simulink model "pocketcorr"  (Simulink 6.2)
settings: Solver=ode45  StartTime=0.0  StopTime=500  RelTol=1e-3
libraries: xbsIndex_r3 x44, xps_library x4, fft_library x4, pfb_library x4, correlator_library x1
settings Model: LastModifiedBy=dejesusc
settings DebuggingCC: SolverPrmCheckMsg=warning

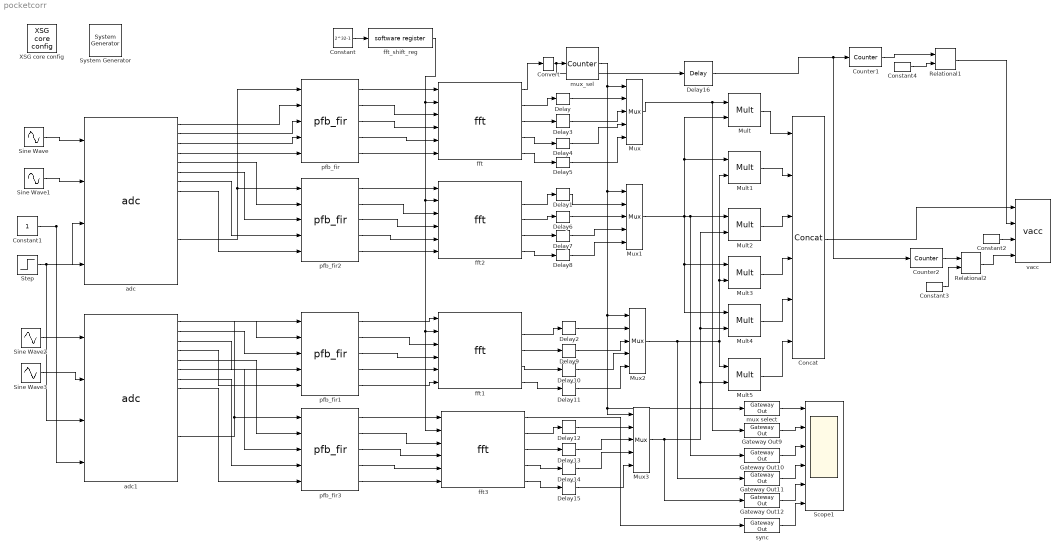
== system pocketcorr ==
  " System Generator" : xbsIndex_r3/ System Generator  Tag=genX  xilinxfamily=Virtex2P  part=xc2vp50  speed=-7  package=ff1152  synthesis_tool=XST  directory=./pocketcorr/sysgen  testbench=off  simulink_period=1  sysclk_period=3.9063  incr_netlist=off  trim_vbits=Everywhere in SubSystem  dbl_ovrd=According to Block Masks  core_generation=According to Block Masks  run_coregen=off  deprecated_control=off  eval_field=0
      settings: AttributesFormatString=System\nGenerator
  Concat : xbsIndex_r3/Concat  num_inputs=6  explicit_period=off  period=1  dbl_ovrd=off
  Constant : Constant  Value=2^32-1
  Constant1 : Constant
  Constant2 : xbsIndex_r3/Constant  const=0  equ=P=C  arith_type=Boolean  n_bits=1  bin_pt=0  opselect=C  inp2=PCIN>>17  opr=+  inp1=P  carry=CIN  iostate=0  explicit_period=on  period=1  dbl_ovrd=off
  Constant3 : xbsIndex_r3/Constant  const=32  equ=P=C  arith_type=Unsigned  n_bits=5  bin_pt=0  opselect=C  inp2=PCIN>>17  opr=+  inp1=P  carry=CIN  iostate=0  explicit_period=on  period=1  dbl_ovrd=off
  Constant4 : xbsIndex_r3/Constant  const=2^4  equ=P=C  arith_type=Unsigned  n_bits=5  bin_pt=0  opselect=C  inp2=PCIN>>17  opr=+  inp1=P  carry=CIN  iostate=0  explicit_period=on  period=1  dbl_ovrd=off
  Convert : xbsIndex_r3/Convert  arith_type=Boolean  n_bits=8  bin_pt=6  quantization=Truncate  overflow=Wrap  latency=0  explicit_period=off  period=1  dbl_ovrd=off  show_param=off  inserted_by_tool=off  pipeline=off
      settings: xl_area=[0, 0, 0, 0, 0, 0, 0]
  Counter1 : xbsIndex_r3/Counter  cnt_type=Free Running  n_bits=5  bin_pt=0  arith_type=Unsigned  start_count=0  cnt_to=Inf  cnt_by_val=1  operation=Up  explicit_period=off  period=1  load_pin=off  rst=on  en=off  dbl_ovrd=off  show_param=off  use_rpm=on  gen_core=off
      settings: xl_area=[0, 0, 0, 0, 0, 0, 0]
  Counter2 : xbsIndex_r3/Counter  cnt_type=Free Running  n_bits=20  bin_pt=0  arith_type=Unsigned  start_count=0  cnt_to=Inf  cnt_by_val=1  operation=Up  explicit_period=off  period=1  load_pin=off  rst=on  en=off  dbl_ovrd=off  show_param=off  use_rpm=on  gen_core=off
      settings: xl_area=[0, 0, 0, 0, 0, 0, 0]
  Delay{,1..2,12} (4 alike) : xbsIndex_r3/Delay  latency=4  reg_retiming=off  explicit_period=off  period=1  en=off  accept_only_valid=off  init_zero=on  dbl_ovrd=off  show_param=off
      settings: xl_area=[0, 0, 0, 0, 0, 0, 0]
  Delay{4,7,10,14} (4 alike) : xbsIndex_r3/Delay  latency=6  reg_retiming=off  explicit_period=off  period=1  en=off  accept_only_valid=off  init_zero=on  dbl_ovrd=off  show_param=off
      settings: xl_area=[0, 0, 0, 0, 0, 0, 0]
  Delay{5,8,11,15} (4 alike) : xbsIndex_r3/Delay  latency=7  reg_retiming=off  explicit_period=off  period=1  en=off  accept_only_valid=off  init_zero=on  dbl_ovrd=off  show_param=off
      settings: xl_area=[0, 0, 0, 0, 0, 0, 0]
  Delay{3,6,9,13} (4 alike) : xbsIndex_r3/Delay  latency=5  reg_retiming=off  explicit_period=off  period=1  en=off  accept_only_valid=off  init_zero=on  dbl_ovrd=off  show_param=off
      settings: xl_area=[0, 0, 0, 0, 0, 0, 0]
  Delay16 : xbsIndex_r3/Delay  latency=9  reg_retiming=off  explicit_period=off  period=1  en=off  accept_only_valid=off  init_zero=on  dbl_ovrd=off  show_param=off
      settings: xl_area=[0, 0, 0, 0, 0, 0, 0]
  Gateway Out{9..12} (4 alike) : xbsIndex_r3/Gateway Out  output_type=Double  nbits=8  bin_pt=6  arith_type=Boolean  quantization=Truncate  overflow=Wrap  hdl_port=on  timing_constraint=None  locs_specified=off  LOCs={}  needs_fixed_name=off  show_param=off
      settings: xl_area=[0, 0, 0, 0, 0, 0, 0]
  Mult{,1..5} (6 alike) : xbsIndex_r3/Mult  precision=Full  arith_type="Signed  (2's comp)"  n_bits=8  bin_pt=2  quantization=Truncate  overflow=Wrap  latency=5  explicit_period=off  period=1  en=off  dbl_ovrd=off  show_param=off  mult_type=Parallel  oversample=2  use_embedded=off  pipeline=on  use_rpm=on  placement_style=Rectangular Shape  gen_core=off
      settings: xl_area=[0, 0, 0, 0, 0, 0, 0]
  Mux{,1..3} (4 alike) : xbsIndex_r3/Mux  inputs=4  precision=Full  arith_type="Signed  (2's comp)"  n_bits=8  bin_pt=2  quantization=Truncate  overflow=Wrap  latency=0  explicit_period=off  period=1  en=off  dbl_ovrd=off  show_param=off  mux_type=off  use_rpm=off  gen_core=off
      settings: xl_area=[0, 0, 0, 0, 0, 0, 0]
  Relational1 : xbsIndex_r3/Relational  mode=a<b  latency=1  explicit_period=on  period=1  en=off  dbl_ovrd=off  show_param=off
      settings: xl_area=[0, 0, 0, 0, 0, 0, 0]
  Relational2 : xbsIndex_r3/Relational  mode=a<b  latency=1  explicit_period=on  period=1  en=off  dbl_ovrd=off  show_param=off
      settings: xl_area=[0, 0, 0, 0, 0, 0, 0]
  Scope1 : Scope  NumInputPorts=6
      settings: YMin=-5~-5~-5~-5~-5~-5  YMax=5~5~5~5~5~5
  Sine Wave : Sin  SampleTime=0
  Sine Wave1 : Sin  Phase=pi  SampleTime=0
  Sine Wave2 : Sin  Phase=pi/2  SampleTime=0
  Sine Wave3 : Sin  Phase=3*pi/2  SampleTime=0
  Step : Step  Time=10  Before=1  After=0  SampleTime=0
  XSG core config : xps_library/XSG core config  Tag=xps:xsg  hw_sys=iBOB  clk_src=adc0_clk  clk_rate=256  sample_period=1  probe_depth=512  mpc_type=powerpc405
  adc : xps_library/adc  Tag=xps:adc  adc_brd=iBOB:adc0  adc_clk_rate=1024  adc_interleave=off  sample_period=1
  adc1 : xps_library/adc  Tag=xps:adc  adc_brd=iBOB:adc1  adc_clk_rate=1024  adc_interleave=off  sample_period=1
  fft : fft_library/fft  FFTSize=5  BitWidth=18  n_inputs=2  quantization="Round  (unbiased: Even Values)"  overflow=Wrap  add_latency=2  mult_latency=3  bram_latency=2
      link override fft_biplex0/biplex_core/fft_stage_1/sync_delay_x/Constant: equ=P=C
      link override fft_biplex0/biplex_core/fft_stage_1/sync_delay_x/Constant1: equ=P=C
      link override fft_biplex0/biplex_core/fft_stage_1/sync_delay_x/Constant2: equ=P=C
      link override fft_biplex0/biplex_core/fft_stage_1/sync_delay_x/Constant3: equ=P=C
      link override fft_biplex0/biplex_core/fft_stage_2/sync_delay_x/Constant: equ=P=C
      link override fft_biplex0/biplex_core/fft_stage_2/sync_delay_x/Constant1: equ=P=C
      link override fft_biplex0/biplex_core/fft_stage_2/sync_delay_x/Constant2: equ=P=C
      link override fft_biplex0/biplex_core/fft_stage_2/sync_delay_x/Constant3: equ=P=C
      link override fft_biplex0/biplex_core/fft_stage_3/sync_delay_x/Constant: equ=P=C
      link override fft_biplex0/biplex_core/fft_stage_3/sync_delay_x/Constant1: equ=P=C
      link override fft_biplex0/biplex_core/fft_stage_3/sync_delay_x/Constant2: equ=P=C
      link override fft_biplex0/biplex_core/fft_stage_3/sync_delay_x/Constant3: equ=P=C
      link override fft_biplex0/biplex_core/fft_stage_4/sync_delay_x/Constant: equ=P=C
      link override fft_biplex0/biplex_core/fft_stage_4/sync_delay_x/Constant1: equ=P=C
      link override fft_biplex0/biplex_core/fft_stage_4/sync_delay_x/Constant2: equ=P=C
      link override fft_biplex0/biplex_core/fft_stage_4/sync_delay_x/Constant3: equ=P=C
      link override fft_biplex0/biplex_core/fft_stage_5/sync_delay_x/Constant: equ=P=C
      link override fft_biplex0/biplex_core/fft_stage_5/sync_delay_x/Constant1: equ=P=C
      link override fft_biplex0/biplex_core/fft_stage_5/sync_delay_x/Constant2: equ=P=C
      link override fft_biplex0/biplex_core/fft_stage_5/sync_delay_x/Constant3: equ=P=C
      link override fft_biplex0/biplex_core/fft_stage_6/sync_delay_x/Constant: equ=P=C
      link override fft_biplex0/biplex_core/fft_stage_6/sync_delay_x/Constant1: equ=P=C
      link override fft_biplex0/biplex_core/fft_stage_6/sync_delay_x/Constant2: equ=P=C
      link override fft_biplex0/biplex_core/fft_stage_6/sync_delay_x/Constant3: equ=P=C
      link override fft_biplex0/biplex_core/fft_stage_7/sync_delay_x/Constant: equ=P=C
      link override fft_biplex0/biplex_core/fft_stage_7/sync_delay_x/Constant1: equ=P=C
      link override fft_biplex0/biplex_core/fft_stage_7/sync_delay_x/Constant2: equ=P=C
      link override fft_biplex0/biplex_core/fft_stage_7/sync_delay_x/Constant3: equ=P=C
      link override fft_biplex0/biplex_cplx_unscrambler/delay_bram1/Constant2: equ=P=C
      link override fft_biplex0/biplex_cplx_unscrambler/reorder/Constant: equ=P=C
      link override fft_biplex0/biplex_cplx_unscrambler/reorder/sync_delay/Constant: equ=P=C
      link override fft_biplex0/biplex_cplx_unscrambler/reorder/sync_delay/Constant1: equ=P=C
      link override fft_biplex0/biplex_cplx_unscrambler/reorder/sync_delay/Constant2: equ=P=C
      link override fft_biplex0/biplex_cplx_unscrambler/reorder/sync_delay/Constant3: equ=P=C
      link override fft_biplex0/biplex_cplx_unscrambler/reorder1/Constant: equ=P=C
      link override fft_biplex0/biplex_cplx_unscrambler/reorder1/sync_delay/Constant: equ=P=C
      link override fft_biplex0/biplex_cplx_unscrambler/reorder1/sync_delay/Constant1: equ=P=C
      link override fft_biplex0/biplex_cplx_unscrambler/reorder1/sync_delay/Constant2: equ=P=C
      link override fft_biplex0/biplex_cplx_unscrambler/reorder1/sync_delay/Constant3: equ=P=C
      link override fft_biplex0/biplex_cplx_unscrambler/sync_delay/Constant: equ=P=C
      link override fft_biplex0/biplex_cplx_unscrambler/sync_delay/Constant1: equ=P=C
      link override fft_biplex0/biplex_cplx_unscrambler/sync_delay/Constant2: equ=P=C
      link override fft_biplex0/biplex_cplx_unscrambler/sync_delay/Constant3: equ=P=C
      link override fft_biplex1/biplex_core/fft_stage_1/sync_delay_x/Constant: equ=P=C
      link override fft_biplex1/biplex_core/fft_stage_1/sync_delay_x/Constant1: equ=P=C
      link override fft_biplex1/biplex_core/fft_stage_1/sync_delay_x/Constant2: equ=P=C
      link override fft_biplex1/biplex_core/fft_stage_1/sync_delay_x/Constant3: equ=P=C
      link override fft_biplex1/biplex_core/fft_stage_2/sync_delay_x/Constant: equ=P=C
      link override fft_biplex1/biplex_core/fft_stage_2/sync_delay_x/Constant1: equ=P=C
      link override fft_biplex1/biplex_core/fft_stage_2/sync_delay_x/Constant2: equ=P=C
      link override fft_biplex1/biplex_core/fft_stage_2/sync_delay_x/Constant3: equ=P=C
      link override fft_biplex1/biplex_core/fft_stage_3/sync_delay_x/Constant: equ=P=C
      link override fft_biplex1/biplex_core/fft_stage_3/sync_delay_x/Constant1: equ=P=C
      link override fft_biplex1/biplex_core/fft_stage_3/sync_delay_x/Constant2: equ=P=C
      link override fft_biplex1/biplex_core/fft_stage_3/sync_delay_x/Constant3: equ=P=C
      link override fft_biplex1/biplex_core/fft_stage_4/sync_delay_x/Constant: equ=P=C
      link override fft_biplex1/biplex_core/fft_stage_4/sync_delay_x/Constant1: equ=P=C
      link override fft_biplex1/biplex_core/fft_stage_4/sync_delay_x/Constant2: equ=P=C
      link override fft_biplex1/biplex_core/fft_stage_4/sync_delay_x/Constant3: equ=P=C
      link override fft_biplex1/biplex_core/fft_stage_5/sync_delay_x/Constant: equ=P=C
      link override fft_biplex1/biplex_core/fft_stage_5/sync_delay_x/Constant1: equ=P=C
      link override fft_biplex1/biplex_core/fft_stage_5/sync_delay_x/Constant2: equ=P=C
      link override fft_biplex1/biplex_core/fft_stage_5/sync_delay_x/Constant3: equ=P=C
      link override fft_biplex1/biplex_core/fft_stage_6/sync_delay_x/Constant: equ=P=C
      link override fft_biplex1/biplex_core/fft_stage_6/sync_delay_x/Constant1: equ=P=C
      link override fft_biplex1/biplex_core/fft_stage_6/sync_delay_x/Constant2: equ=P=C
      link override fft_biplex1/biplex_core/fft_stage_6/sync_delay_x/Constant3: equ=P=C
      link override fft_biplex1/biplex_core/fft_stage_7/sync_delay_x/Constant: equ=P=C
      link override fft_biplex1/biplex_core/fft_stage_7/sync_delay_x/Constant1: equ=P=C
      link override fft_biplex1/biplex_core/fft_stage_7/sync_delay_x/Constant2: equ=P=C
      link override fft_biplex1/biplex_core/fft_stage_7/sync_delay_x/Constant3: equ=P=C
      link override fft_biplex1/biplex_cplx_unscrambler/delay_bram1/Constant2: equ=P=C
      link override fft_biplex1/biplex_cplx_unscrambler/reorder/Constant: equ=P=C
      link override fft_biplex1/biplex_cplx_unscrambler/reorder/sync_delay/Constant: equ=P=C
      link override fft_biplex1/biplex_cplx_unscrambler/reorder/sync_delay/Constant1: equ=P=C
      link override fft_biplex1/biplex_cplx_unscrambler/reorder/sync_delay/Constant2: equ=P=C
      link override fft_biplex1/biplex_cplx_unscrambler/reorder/sync_delay/Constant3: equ=P=C
      link override fft_biplex1/biplex_cplx_unscrambler/reorder1/Constant: equ=P=C
      link override fft_biplex1/biplex_cplx_unscrambler/reorder1/sync_delay/Constant: equ=P=C
      link override fft_biplex1/biplex_cplx_unscrambler/reorder1/sync_delay/Constant1: equ=P=C
      link override fft_biplex1/biplex_cplx_unscrambler/reorder1/sync_delay/Constant2: equ=P=C
      link override fft_biplex1/biplex_cplx_unscrambler/reorder1/sync_delay/Constant3: equ=P=C
      link override fft_biplex1/biplex_cplx_unscrambler/sync_delay/Constant: equ=P=C
      link override fft_biplex1/biplex_cplx_unscrambler/sync_delay/Constant1: equ=P=C
      link override fft_biplex1/biplex_cplx_unscrambler/sync_delay/Constant2: equ=P=C
      link override fft_biplex1/biplex_cplx_unscrambler/sync_delay/Constant3: equ=P=C
      link override fft_unscrambler/Constant: const=1  equ=P=C  arith_type=Boolean  explicit_period=on
      link override fft_unscrambler/sync_delay/Constant: equ=P=C
      link override fft_unscrambler/sync_delay/Constant1: equ=P=C
      link override fft_unscrambler/sync_delay/Constant2: equ=P=C
      link override fft_unscrambler/sync_delay/Constant3: equ=P=C
  fft1 : fft_library/fft  FFTSize=5  BitWidth=18  n_inputs=2  quantization="Round  (unbiased: Even Values)"  overflow=Wrap  add_latency=2  mult_latency=3  bram_latency=2
      link override fft_biplex0/biplex_core/fft_stage_1/sync_delay_x/Constant: equ=P=C
      link override fft_biplex0/biplex_core/fft_stage_1/sync_delay_x/Constant1: equ=P=C
      link override fft_biplex0/biplex_core/fft_stage_1/sync_delay_x/Constant2: equ=P=C
      link override fft_biplex0/biplex_core/fft_stage_1/sync_delay_x/Constant3: equ=P=C
      link override fft_biplex0/biplex_core/fft_stage_2/sync_delay_x/Constant: equ=P=C
      link override fft_biplex0/biplex_core/fft_stage_2/sync_delay_x/Constant1: equ=P=C
      link override fft_biplex0/biplex_core/fft_stage_2/sync_delay_x/Constant2: equ=P=C
      link override fft_biplex0/biplex_core/fft_stage_2/sync_delay_x/Constant3: equ=P=C
      link override fft_biplex0/biplex_core/fft_stage_3/sync_delay_x/Constant: equ=P=C
      link override fft_biplex0/biplex_core/fft_stage_3/sync_delay_x/Constant1: equ=P=C
      link override fft_biplex0/biplex_core/fft_stage_3/sync_delay_x/Constant2: equ=P=C
      link override fft_biplex0/biplex_core/fft_stage_3/sync_delay_x/Constant3: equ=P=C
      link override fft_biplex0/biplex_core/fft_stage_4/sync_delay_x/Constant: equ=P=C
      link override fft_biplex0/biplex_core/fft_stage_4/sync_delay_x/Constant1: equ=P=C
      link override fft_biplex0/biplex_core/fft_stage_4/sync_delay_x/Constant2: equ=P=C
      link override fft_biplex0/biplex_core/fft_stage_4/sync_delay_x/Constant3: equ=P=C
      link override fft_biplex0/biplex_core/fft_stage_5/sync_delay_x/Constant: equ=P=C
      link override fft_biplex0/biplex_core/fft_stage_5/sync_delay_x/Constant1: equ=P=C
      link override fft_biplex0/biplex_core/fft_stage_5/sync_delay_x/Constant2: equ=P=C
      link override fft_biplex0/biplex_core/fft_stage_5/sync_delay_x/Constant3: equ=P=C
      link override fft_biplex0/biplex_core/fft_stage_6/sync_delay_x/Constant: equ=P=C
      link override fft_biplex0/biplex_core/fft_stage_6/sync_delay_x/Constant1: equ=P=C
      link override fft_biplex0/biplex_core/fft_stage_6/sync_delay_x/Constant2: equ=P=C
      link override fft_biplex0/biplex_core/fft_stage_6/sync_delay_x/Constant3: equ=P=C
      link override fft_biplex0/biplex_core/fft_stage_7/sync_delay_x/Constant: equ=P=C
      link override fft_biplex0/biplex_core/fft_stage_7/sync_delay_x/Constant1: equ=P=C
      link override fft_biplex0/biplex_core/fft_stage_7/sync_delay_x/Constant2: equ=P=C
      link override fft_biplex0/biplex_core/fft_stage_7/sync_delay_x/Constant3: equ=P=C
      link override fft_biplex0/biplex_cplx_unscrambler/delay_bram1/Constant2: equ=P=C
      link override fft_biplex0/biplex_cplx_unscrambler/reorder/Constant: equ=P=C
      link override fft_biplex0/biplex_cplx_unscrambler/reorder/sync_delay/Constant: equ=P=C
      link override fft_biplex0/biplex_cplx_unscrambler/reorder/sync_delay/Constant1: equ=P=C
      link override fft_biplex0/biplex_cplx_unscrambler/reorder/sync_delay/Constant2: equ=P=C
      link override fft_biplex0/biplex_cplx_unscrambler/reorder/sync_delay/Constant3: equ=P=C
      link override fft_biplex0/biplex_cplx_unscrambler/reorder1/Constant: equ=P=C
      link override fft_biplex0/biplex_cplx_unscrambler/reorder1/sync_delay/Constant: equ=P=C
      link override fft_biplex0/biplex_cplx_unscrambler/reorder1/sync_delay/Constant1: equ=P=C
      link override fft_biplex0/biplex_cplx_unscrambler/reorder1/sync_delay/Constant2: equ=P=C
      link override fft_biplex0/biplex_cplx_unscrambler/reorder1/sync_delay/Constant3: equ=P=C
      link override fft_biplex0/biplex_cplx_unscrambler/sync_delay/Constant: equ=P=C
      link override fft_biplex0/biplex_cplx_unscrambler/sync_delay/Constant1: equ=P=C
      link override fft_biplex0/biplex_cplx_unscrambler/sync_delay/Constant2: equ=P=C
      link override fft_biplex0/biplex_cplx_unscrambler/sync_delay/Constant3: equ=P=C
      link override fft_biplex1/biplex_core/fft_stage_1/sync_delay_x/Constant: equ=P=C
      link override fft_biplex1/biplex_core/fft_stage_1/sync_delay_x/Constant1: equ=P=C
      link override fft_biplex1/biplex_core/fft_stage_1/sync_delay_x/Constant2: equ=P=C
      link override fft_biplex1/biplex_core/fft_stage_1/sync_delay_x/Constant3: equ=P=C
      link override fft_biplex1/biplex_core/fft_stage_2/sync_delay_x/Constant: equ=P=C
      link override fft_biplex1/biplex_core/fft_stage_2/sync_delay_x/Constant1: equ=P=C
      link override fft_biplex1/biplex_core/fft_stage_2/sync_delay_x/Constant2: equ=P=C
      link override fft_biplex1/biplex_core/fft_stage_2/sync_delay_x/Constant3: equ=P=C
      link override fft_biplex1/biplex_core/fft_stage_3/sync_delay_x/Constant: equ=P=C
      link override fft_biplex1/biplex_core/fft_stage_3/sync_delay_x/Constant1: equ=P=C
      link override fft_biplex1/biplex_core/fft_stage_3/sync_delay_x/Constant2: equ=P=C
      link override fft_biplex1/biplex_core/fft_stage_3/sync_delay_x/Constant3: equ=P=C
      link override fft_biplex1/biplex_core/fft_stage_4/sync_delay_x/Constant: equ=P=C
      link override fft_biplex1/biplex_core/fft_stage_4/sync_delay_x/Constant1: equ=P=C
      link override fft_biplex1/biplex_core/fft_stage_4/sync_delay_x/Constant2: equ=P=C
      link override fft_biplex1/biplex_core/fft_stage_4/sync_delay_x/Constant3: equ=P=C
      link override fft_biplex1/biplex_core/fft_stage_5/sync_delay_x/Constant: equ=P=C
      link override fft_biplex1/biplex_core/fft_stage_5/sync_delay_x/Constant1: equ=P=C
      link override fft_biplex1/biplex_core/fft_stage_5/sync_delay_x/Constant2: equ=P=C
      link override fft_biplex1/biplex_core/fft_stage_5/sync_delay_x/Constant3: equ=P=C
      link override fft_biplex1/biplex_core/fft_stage_6/sync_delay_x/Constant: equ=P=C
      link override fft_biplex1/biplex_core/fft_stage_6/sync_delay_x/Constant1: equ=P=C
      link override fft_biplex1/biplex_core/fft_stage_6/sync_delay_x/Constant2: equ=P=C
      link override fft_biplex1/biplex_core/fft_stage_6/sync_delay_x/Constant3: equ=P=C
      link override fft_biplex1/biplex_core/fft_stage_7/sync_delay_x/Constant: equ=P=C
      link override fft_biplex1/biplex_core/fft_stage_7/sync_delay_x/Constant1: equ=P=C
      link override fft_biplex1/biplex_core/fft_stage_7/sync_delay_x/Constant2: equ=P=C
      link override fft_biplex1/biplex_core/fft_stage_7/sync_delay_x/Constant3: equ=P=C
      link override fft_biplex1/biplex_cplx_unscrambler/delay_bram1/Constant2: equ=P=C
      link override fft_biplex1/biplex_cplx_unscrambler/reorder/Constant: equ=P=C
      link override fft_biplex1/biplex_cplx_unscrambler/reorder/sync_delay/Constant: equ=P=C
      link override fft_biplex1/biplex_cplx_unscrambler/reorder/sync_delay/Constant1: equ=P=C
      link override fft_biplex1/biplex_cplx_unscrambler/reorder/sync_delay/Constant2: equ=P=C
      link override fft_biplex1/biplex_cplx_unscrambler/reorder/sync_delay/Constant3: equ=P=C
      link override fft_biplex1/biplex_cplx_unscrambler/reorder1/Constant: equ=P=C
      link override fft_biplex1/biplex_cplx_unscrambler/reorder1/sync_delay/Constant: equ=P=C
      link override fft_biplex1/biplex_cplx_unscrambler/reorder1/sync_delay/Constant1: equ=P=C
      link override fft_biplex1/biplex_cplx_unscrambler/reorder1/sync_delay/Constant2: equ=P=C
      link override fft_biplex1/biplex_cplx_unscrambler/reorder1/sync_delay/Constant3: equ=P=C
      link override fft_biplex1/biplex_cplx_unscrambler/sync_delay/Constant: equ=P=C
      link override fft_biplex1/biplex_cplx_unscrambler/sync_delay/Constant1: equ=P=C
      link override fft_biplex1/biplex_cplx_unscrambler/sync_delay/Constant2: equ=P=C
      link override fft_biplex1/biplex_cplx_unscrambler/sync_delay/Constant3: equ=P=C
      link override fft_unscrambler/Constant: equ=P=C  const=1  arith_type=Boolean  explicit_period=on
      link override fft_unscrambler/sync_delay/Constant: equ=P=C
      link override fft_unscrambler/sync_delay/Constant1: equ=P=C
      link override fft_unscrambler/sync_delay/Constant2: equ=P=C
      link override fft_unscrambler/sync_delay/Constant3: equ=P=C
  fft2 : fft_library/fft  FFTSize=5  BitWidth=18  n_inputs=2  quantization="Round  (unbiased: Even Values)"  overflow=Wrap  add_latency=2  mult_latency=3  bram_latency=2
      link override fft_biplex0/biplex_core/fft_stage_1/sync_delay_x/Constant: equ=P=C
      link override fft_biplex0/biplex_core/fft_stage_1/sync_delay_x/Constant1: equ=P=C
      link override fft_biplex0/biplex_core/fft_stage_1/sync_delay_x/Constant2: equ=P=C
      link override fft_biplex0/biplex_core/fft_stage_1/sync_delay_x/Constant3: equ=P=C
      link override fft_biplex0/biplex_core/fft_stage_2/sync_delay_x/Constant: equ=P=C
      link override fft_biplex0/biplex_core/fft_stage_2/sync_delay_x/Constant1: equ=P=C
      link override fft_biplex0/biplex_core/fft_stage_2/sync_delay_x/Constant2: equ=P=C
      link override fft_biplex0/biplex_core/fft_stage_2/sync_delay_x/Constant3: equ=P=C
      link override fft_biplex0/biplex_core/fft_stage_3/sync_delay_x/Constant: equ=P=C
      link override fft_biplex0/biplex_core/fft_stage_3/sync_delay_x/Constant1: equ=P=C
      link override fft_biplex0/biplex_core/fft_stage_3/sync_delay_x/Constant2: equ=P=C
      link override fft_biplex0/biplex_core/fft_stage_3/sync_delay_x/Constant3: equ=P=C
      link override fft_biplex0/biplex_core/fft_stage_4/sync_delay_x/Constant: equ=P=C
      link override fft_biplex0/biplex_core/fft_stage_4/sync_delay_x/Constant1: equ=P=C
      link override fft_biplex0/biplex_core/fft_stage_4/sync_delay_x/Constant2: equ=P=C
      link override fft_biplex0/biplex_core/fft_stage_4/sync_delay_x/Constant3: equ=P=C
      link override fft_biplex0/biplex_core/fft_stage_5/sync_delay_x/Constant: equ=P=C
      link override fft_biplex0/biplex_core/fft_stage_5/sync_delay_x/Constant1: equ=P=C
      link override fft_biplex0/biplex_core/fft_stage_5/sync_delay_x/Constant2: equ=P=C
      link override fft_biplex0/biplex_core/fft_stage_5/sync_delay_x/Constant3: equ=P=C
      link override fft_biplex0/biplex_core/fft_stage_6/sync_delay_x/Constant: equ=P=C
      link override fft_biplex0/biplex_core/fft_stage_6/sync_delay_x/Constant1: equ=P=C
      link override fft_biplex0/biplex_core/fft_stage_6/sync_delay_x/Constant2: equ=P=C
      link override fft_biplex0/biplex_core/fft_stage_6/sync_delay_x/Constant3: equ=P=C
      link override fft_biplex0/biplex_core/fft_stage_7/sync_delay_x/Constant: equ=P=C
      link override fft_biplex0/biplex_core/fft_stage_7/sync_delay_x/Constant1: equ=P=C
      link override fft_biplex0/biplex_core/fft_stage_7/sync_delay_x/Constant2: equ=P=C
      link override fft_biplex0/biplex_core/fft_stage_7/sync_delay_x/Constant3: equ=P=C
      link override fft_biplex0/biplex_cplx_unscrambler/delay_bram1/Constant2: equ=P=C
      link override fft_biplex0/biplex_cplx_unscrambler/reorder/Constant: equ=P=C
      link override fft_biplex0/biplex_cplx_unscrambler/reorder/sync_delay/Constant: equ=P=C
      link override fft_biplex0/biplex_cplx_unscrambler/reorder/sync_delay/Constant1: equ=P=C
      link override fft_biplex0/biplex_cplx_unscrambler/reorder/sync_delay/Constant2: equ=P=C
      link override fft_biplex0/biplex_cplx_unscrambler/reorder/sync_delay/Constant3: equ=P=C
      link override fft_biplex0/biplex_cplx_unscrambler/reorder1/Constant: equ=P=C
      link override fft_biplex0/biplex_cplx_unscrambler/reorder1/sync_delay/Constant: equ=P=C
      link override fft_biplex0/biplex_cplx_unscrambler/reorder1/sync_delay/Constant1: equ=P=C
      link override fft_biplex0/biplex_cplx_unscrambler/reorder1/sync_delay/Constant2: equ=P=C
      link override fft_biplex0/biplex_cplx_unscrambler/reorder1/sync_delay/Constant3: equ=P=C
      link override fft_biplex0/biplex_cplx_unscrambler/sync_delay/Constant: equ=P=C
      link override fft_biplex0/biplex_cplx_unscrambler/sync_delay/Constant1: equ=P=C
      link override fft_biplex0/biplex_cplx_unscrambler/sync_delay/Constant2: equ=P=C
      link override fft_biplex0/biplex_cplx_unscrambler/sync_delay/Constant3: equ=P=C
      link override fft_biplex1/biplex_core/fft_stage_1/sync_delay_x/Constant: equ=P=C
      link override fft_biplex1/biplex_core/fft_stage_1/sync_delay_x/Constant1: equ=P=C
      link override fft_biplex1/biplex_core/fft_stage_1/sync_delay_x/Constant2: equ=P=C
      link override fft_biplex1/biplex_core/fft_stage_1/sync_delay_x/Constant3: equ=P=C
      link override fft_biplex1/biplex_core/fft_stage_2/sync_delay_x/Constant: equ=P=C
      link override fft_biplex1/biplex_core/fft_stage_2/sync_delay_x/Constant1: equ=P=C
      link override fft_biplex1/biplex_core/fft_stage_2/sync_delay_x/Constant2: equ=P=C
      link override fft_biplex1/biplex_core/fft_stage_2/sync_delay_x/Constant3: equ=P=C
      link override fft_biplex1/biplex_core/fft_stage_3/sync_delay_x/Constant: equ=P=C
      link override fft_biplex1/biplex_core/fft_stage_3/sync_delay_x/Constant1: equ=P=C
      link override fft_biplex1/biplex_core/fft_stage_3/sync_delay_x/Constant2: equ=P=C
      link override fft_biplex1/biplex_core/fft_stage_3/sync_delay_x/Constant3: equ=P=C
      link override fft_biplex1/biplex_core/fft_stage_4/sync_delay_x/Constant: equ=P=C
      link override fft_biplex1/biplex_core/fft_stage_4/sync_delay_x/Constant1: equ=P=C
      link override fft_biplex1/biplex_core/fft_stage_4/sync_delay_x/Constant2: equ=P=C
      link override fft_biplex1/biplex_core/fft_stage_4/sync_delay_x/Constant3: equ=P=C
      link override fft_biplex1/biplex_core/fft_stage_5/sync_delay_x/Constant: equ=P=C
      link override fft_biplex1/biplex_core/fft_stage_5/sync_delay_x/Constant1: equ=P=C
      link override fft_biplex1/biplex_core/fft_stage_5/sync_delay_x/Constant2: equ=P=C
      link override fft_biplex1/biplex_core/fft_stage_5/sync_delay_x/Constant3: equ=P=C
      link override fft_biplex1/biplex_core/fft_stage_6/sync_delay_x/Constant: equ=P=C
      link override fft_biplex1/biplex_core/fft_stage_6/sync_delay_x/Constant1: equ=P=C
      link override fft_biplex1/biplex_core/fft_stage_6/sync_delay_x/Constant2: equ=P=C
      link override fft_biplex1/biplex_core/fft_stage_6/sync_delay_x/Constant3: equ=P=C
      link override fft_biplex1/biplex_core/fft_stage_7/sync_delay_x/Constant: equ=P=C
      link override fft_biplex1/biplex_core/fft_stage_7/sync_delay_x/Constant1: equ=P=C
      link override fft_biplex1/biplex_core/fft_stage_7/sync_delay_x/Constant2: equ=P=C
      link override fft_biplex1/biplex_core/fft_stage_7/sync_delay_x/Constant3: equ=P=C
      link override fft_biplex1/biplex_cplx_unscrambler/delay_bram1/Constant2: equ=P=C
      link override fft_biplex1/biplex_cplx_unscrambler/reorder/Constant: equ=P=C
      link override fft_biplex1/biplex_cplx_unscrambler/reorder/sync_delay/Constant: equ=P=C
      link override fft_biplex1/biplex_cplx_unscrambler/reorder/sync_delay/Constant1: equ=P=C
      link override fft_biplex1/biplex_cplx_unscrambler/reorder/sync_delay/Constant2: equ=P=C
      link override fft_biplex1/biplex_cplx_unscrambler/reorder/sync_delay/Constant3: equ=P=C
      link override fft_biplex1/biplex_cplx_unscrambler/reorder1/Constant: equ=P=C
      link override fft_biplex1/biplex_cplx_unscrambler/reorder1/sync_delay/Constant: equ=P=C
      link override fft_biplex1/biplex_cplx_unscrambler/reorder1/sync_delay/Constant1: equ=P=C
      link override fft_biplex1/biplex_cplx_unscrambler/reorder1/sync_delay/Constant2: equ=P=C
      link override fft_biplex1/biplex_cplx_unscrambler/reorder1/sync_delay/Constant3: equ=P=C
      link override fft_biplex1/biplex_cplx_unscrambler/sync_delay/Constant: equ=P=C
      link override fft_biplex1/biplex_cplx_unscrambler/sync_delay/Constant1: equ=P=C
      link override fft_biplex1/biplex_cplx_unscrambler/sync_delay/Constant2: equ=P=C
      link override fft_biplex1/biplex_cplx_unscrambler/sync_delay/Constant3: equ=P=C
      link override fft_unscrambler/Constant: equ=P=C  const=1  arith_type=Boolean  explicit_period=on
      link override fft_unscrambler/sync_delay/Constant: equ=P=C
      link override fft_unscrambler/sync_delay/Constant1: equ=P=C
      link override fft_unscrambler/sync_delay/Constant2: equ=P=C
      link override fft_unscrambler/sync_delay/Constant3: equ=P=C
  fft3 : fft_library/fft  FFTSize=5  BitWidth=18  n_inputs=2  quantization="Round  (unbiased: Even Values)"  overflow=Wrap  add_latency=2  mult_latency=3  bram_latency=2
      link override fft_biplex0/biplex_core/fft_stage_1/sync_delay_x/Constant: equ=P=C
      link override fft_biplex0/biplex_core/fft_stage_1/sync_delay_x/Constant1: equ=P=C
      link override fft_biplex0/biplex_core/fft_stage_1/sync_delay_x/Constant2: equ=P=C
      link override fft_biplex0/biplex_core/fft_stage_1/sync_delay_x/Constant3: equ=P=C
      link override fft_biplex0/biplex_core/fft_stage_2/sync_delay_x/Constant: equ=P=C
      link override fft_biplex0/biplex_core/fft_stage_2/sync_delay_x/Constant1: equ=P=C
      link override fft_biplex0/biplex_core/fft_stage_2/sync_delay_x/Constant2: equ=P=C
      link override fft_biplex0/biplex_core/fft_stage_2/sync_delay_x/Constant3: equ=P=C
      link override fft_biplex0/biplex_core/fft_stage_3/sync_delay_x/Constant: equ=P=C
      link override fft_biplex0/biplex_core/fft_stage_3/sync_delay_x/Constant1: equ=P=C
      link override fft_biplex0/biplex_core/fft_stage_3/sync_delay_x/Constant2: equ=P=C
      link override fft_biplex0/biplex_core/fft_stage_3/sync_delay_x/Constant3: equ=P=C
      link override fft_biplex0/biplex_core/fft_stage_4/sync_delay_x/Constant: equ=P=C
      link override fft_biplex0/biplex_core/fft_stage_4/sync_delay_x/Constant1: equ=P=C
      link override fft_biplex0/biplex_core/fft_stage_4/sync_delay_x/Constant2: equ=P=C
      link override fft_biplex0/biplex_core/fft_stage_4/sync_delay_x/Constant3: equ=P=C
      link override fft_biplex0/biplex_core/fft_stage_5/sync_delay_x/Constant: equ=P=C
      link override fft_biplex0/biplex_core/fft_stage_5/sync_delay_x/Constant1: equ=P=C
      link override fft_biplex0/biplex_core/fft_stage_5/sync_delay_x/Constant2: equ=P=C
      link override fft_biplex0/biplex_core/fft_stage_5/sync_delay_x/Constant3: equ=P=C
      link override fft_biplex0/biplex_core/fft_stage_6/sync_delay_x/Constant: equ=P=C
      link override fft_biplex0/biplex_core/fft_stage_6/sync_delay_x/Constant1: equ=P=C
      link override fft_biplex0/biplex_core/fft_stage_6/sync_delay_x/Constant2: equ=P=C
      link override fft_biplex0/biplex_core/fft_stage_6/sync_delay_x/Constant3: equ=P=C
      link override fft_biplex0/biplex_core/fft_stage_7/sync_delay_x/Constant: equ=P=C
      link override fft_biplex0/biplex_core/fft_stage_7/sync_delay_x/Constant1: equ=P=C
      link override fft_biplex0/biplex_core/fft_stage_7/sync_delay_x/Constant2: equ=P=C
      link override fft_biplex0/biplex_core/fft_stage_7/sync_delay_x/Constant3: equ=P=C
      link override fft_biplex0/biplex_cplx_unscrambler/delay_bram1/Constant2: equ=P=C
      link override fft_biplex0/biplex_cplx_unscrambler/reorder/Constant: equ=P=C
      link override fft_biplex0/biplex_cplx_unscrambler/reorder/sync_delay/Constant: equ=P=C
      link override fft_biplex0/biplex_cplx_unscrambler/reorder/sync_delay/Constant1: equ=P=C
      link override fft_biplex0/biplex_cplx_unscrambler/reorder/sync_delay/Constant2: equ=P=C
      link override fft_biplex0/biplex_cplx_unscrambler/reorder/sync_delay/Constant3: equ=P=C
      link override fft_biplex0/biplex_cplx_unscrambler/reorder1/Constant: equ=P=C
      link override fft_biplex0/biplex_cplx_unscrambler/reorder1/sync_delay/Constant: equ=P=C
      link override fft_biplex0/biplex_cplx_unscrambler/reorder1/sync_delay/Constant1: equ=P=C
      link override fft_biplex0/biplex_cplx_unscrambler/reorder1/sync_delay/Constant2: equ=P=C
      link override fft_biplex0/biplex_cplx_unscrambler/reorder1/sync_delay/Constant3: equ=P=C
      link override fft_biplex0/biplex_cplx_unscrambler/sync_delay/Constant: equ=P=C
      link override fft_biplex0/biplex_cplx_unscrambler/sync_delay/Constant1: equ=P=C
      link override fft_biplex0/biplex_cplx_unscrambler/sync_delay/Constant2: equ=P=C
      link override fft_biplex0/biplex_cplx_unscrambler/sync_delay/Constant3: equ=P=C
      link override fft_biplex1/biplex_core/fft_stage_1/sync_delay_x/Constant: equ=P=C
      link override fft_biplex1/biplex_core/fft_stage_1/sync_delay_x/Constant1: equ=P=C
      link override fft_biplex1/biplex_core/fft_stage_1/sync_delay_x/Constant2: equ=P=C
      link override fft_biplex1/biplex_core/fft_stage_1/sync_delay_x/Constant3: equ=P=C
      link override fft_biplex1/biplex_core/fft_stage_2/sync_delay_x/Constant: equ=P=C
      link override fft_biplex1/biplex_core/fft_stage_2/sync_delay_x/Constant1: equ=P=C
      link override fft_biplex1/biplex_core/fft_stage_2/sync_delay_x/Constant2: equ=P=C
      link override fft_biplex1/biplex_core/fft_stage_2/sync_delay_x/Constant3: equ=P=C
      link override fft_biplex1/biplex_core/fft_stage_3/sync_delay_x/Constant: equ=P=C
      link override fft_biplex1/biplex_core/fft_stage_3/sync_delay_x/Constant1: equ=P=C
      link override fft_biplex1/biplex_core/fft_stage_3/sync_delay_x/Constant2: equ=P=C
      link override fft_biplex1/biplex_core/fft_stage_3/sync_delay_x/Constant3: equ=P=C
      link override fft_biplex1/biplex_core/fft_stage_4/sync_delay_x/Constant: equ=P=C
      link override fft_biplex1/biplex_core/fft_stage_4/sync_delay_x/Constant1: equ=P=C
      link override fft_biplex1/biplex_core/fft_stage_4/sync_delay_x/Constant2: equ=P=C
      link override fft_biplex1/biplex_core/fft_stage_4/sync_delay_x/Constant3: equ=P=C
      link override fft_biplex1/biplex_core/fft_stage_5/sync_delay_x/Constant: equ=P=C
      link override fft_biplex1/biplex_core/fft_stage_5/sync_delay_x/Constant1: equ=P=C
      link override fft_biplex1/biplex_core/fft_stage_5/sync_delay_x/Constant2: equ=P=C
      link override fft_biplex1/biplex_core/fft_stage_5/sync_delay_x/Constant3: equ=P=C
      link override fft_biplex1/biplex_core/fft_stage_6/sync_delay_x/Constant: equ=P=C
      link override fft_biplex1/biplex_core/fft_stage_6/sync_delay_x/Constant1: equ=P=C
      link override fft_biplex1/biplex_core/fft_stage_6/sync_delay_x/Constant2: equ=P=C
      link override fft_biplex1/biplex_core/fft_stage_6/sync_delay_x/Constant3: equ=P=C
      link override fft_biplex1/biplex_core/fft_stage_7/sync_delay_x/Constant: equ=P=C
      link override fft_biplex1/biplex_core/fft_stage_7/sync_delay_x/Constant1: equ=P=C
      link override fft_biplex1/biplex_core/fft_stage_7/sync_delay_x/Constant2: equ=P=C
      link override fft_biplex1/biplex_core/fft_stage_7/sync_delay_x/Constant3: equ=P=C
      link override fft_biplex1/biplex_cplx_unscrambler/delay_bram1/Constant2: equ=P=C
      link override fft_biplex1/biplex_cplx_unscrambler/reorder/Constant: equ=P=C
      link override fft_biplex1/biplex_cplx_unscrambler/reorder/sync_delay/Constant: equ=P=C
      link override fft_biplex1/biplex_cplx_unscrambler/reorder/sync_delay/Constant1: equ=P=C
      link override fft_biplex1/biplex_cplx_unscrambler/reorder/sync_delay/Constant2: equ=P=C
      link override fft_biplex1/biplex_cplx_unscrambler/reorder/sync_delay/Constant3: equ=P=C
      link override fft_biplex1/biplex_cplx_unscrambler/reorder1/Constant: equ=P=C
      link override fft_biplex1/biplex_cplx_unscrambler/reorder1/sync_delay/Constant: equ=P=C
      link override fft_biplex1/biplex_cplx_unscrambler/reorder1/sync_delay/Constant1: equ=P=C
      link override fft_biplex1/biplex_cplx_unscrambler/reorder1/sync_delay/Constant2: equ=P=C
      link override fft_biplex1/biplex_cplx_unscrambler/reorder1/sync_delay/Constant3: equ=P=C
      link override fft_biplex1/biplex_cplx_unscrambler/sync_delay/Constant: equ=P=C
      link override fft_biplex1/biplex_cplx_unscrambler/sync_delay/Constant1: equ=P=C
      link override fft_biplex1/biplex_cplx_unscrambler/sync_delay/Constant2: equ=P=C
      link override fft_biplex1/biplex_cplx_unscrambler/sync_delay/Constant3: equ=P=C
      link override fft_unscrambler/Constant: equ=P=C  const=1  arith_type=Boolean  explicit_period=on
      link override fft_unscrambler/sync_delay/Constant: equ=P=C
      link override fft_unscrambler/sync_delay/Constant1: equ=P=C
      link override fft_unscrambler/sync_delay/Constant2: equ=P=C
      link override fft_unscrambler/sync_delay/Constant3: equ=P=C
  fft_shift_reg : xps_library/software register  Tag=xps:sw_reg  io_dir=From Processor  arith_type=Unsigned  bitwidth=32  bin_pt=0  sample_period=1  gw_name=pocketcorr_fft_shift_reg_user_data_out
  mux select : xbsIndex_r3/Gateway Out  output_type=Double  nbits=8  bin_pt=6  arith_type=Boolean  quantization=Truncate  overflow=Wrap  hdl_port=on  timing_constraint=None  locs_specified=off  LOCs={}  needs_fixed_name=off  show_param=off
      settings: xl_area=[0, 0, 0, 0, 0, 0, 0]
  mux_sel : xbsIndex_r3/Counter  cnt_type=Free Running  n_bits=2  bin_pt=0  arith_type=Unsigned  start_count=0  cnt_to=3  cnt_by_val=1  operation=Up  explicit_period=off  period=1  load_pin=off  rst=on  en=off  dbl_ovrd=off  show_param=off  use_rpm=on  gen_core=off
      settings: xl_area=[0, 0, 0, 0, 0, 0, 0]
  pfb_fir : pfb_library/pfb_fir  PFBSize=5  TotalTaps=2  WindowType=hamming  n_inputs=2  MakeBiplex=off  BitWidthIn=8  BitWidthOut=18  CoeffBitWidth=8  CoeffDistMem=off  add_latency=2  mult_latency=3  bram_latency=2  quantization="Round  (unbiased: +/- Inf)"  fwidth=1
      link override pol1_in1_first_tap/sync_delay/Constant: equ=P=C
      link override pol1_in1_first_tap/sync_delay/Constant1: equ=P=C
      link override pol1_in1_first_tap/sync_delay/Constant2: equ=P=C
      link override pol1_in1_first_tap/sync_delay/Constant3: equ=P=C
      link override pol1_in2_first_tap/sync_delay/Constant: equ=P=C
      link override pol1_in2_first_tap/sync_delay/Constant1: equ=P=C
      link override pol1_in2_first_tap/sync_delay/Constant2: equ=P=C
      link override pol1_in2_first_tap/sync_delay/Constant3: equ=P=C
      link override pol1_in3_first_tap/sync_delay/Constant: equ=P=C
      link override pol1_in3_first_tap/sync_delay/Constant1: equ=P=C
      link override pol1_in3_first_tap/sync_delay/Constant2: equ=P=C
      link override pol1_in3_first_tap/sync_delay/Constant3: equ=P=C
      link override pol1_in4_first_tap/sync_delay/Constant: equ=P=C
      link override pol1_in4_first_tap/sync_delay/Constant1: equ=P=C
      link override pol1_in4_first_tap/sync_delay/Constant2: equ=P=C
      link override pol1_in4_first_tap/sync_delay/Constant3: equ=P=C
  pfb_fir1 : pfb_library/pfb_fir  PFBSize=5  TotalTaps=2  WindowType=hamming  n_inputs=2  MakeBiplex=off  BitWidthIn=8  BitWidthOut=18  CoeffBitWidth=8  CoeffDistMem=off  add_latency=2  mult_latency=3  bram_latency=2  quantization="Round  (unbiased: +/- Inf)"  fwidth=1
      link override pol1_in1_first_tap/sync_delay/Constant: equ=P=C
      link override pol1_in1_first_tap/sync_delay/Constant1: equ=P=C
      link override pol1_in1_first_tap/sync_delay/Constant2: equ=P=C
      link override pol1_in1_first_tap/sync_delay/Constant3: equ=P=C
      link override pol1_in2_first_tap/sync_delay/Constant: equ=P=C
      link override pol1_in2_first_tap/sync_delay/Constant1: equ=P=C
      link override pol1_in2_first_tap/sync_delay/Constant2: equ=P=C
      link override pol1_in2_first_tap/sync_delay/Constant3: equ=P=C
      link override pol1_in3_first_tap/sync_delay/Constant: equ=P=C
      link override pol1_in3_first_tap/sync_delay/Constant1: equ=P=C
      link override pol1_in3_first_tap/sync_delay/Constant2: equ=P=C
      link override pol1_in3_first_tap/sync_delay/Constant3: equ=P=C
      link override pol1_in4_first_tap/sync_delay/Constant: equ=P=C
      link override pol1_in4_first_tap/sync_delay/Constant1: equ=P=C
      link override pol1_in4_first_tap/sync_delay/Constant2: equ=P=C
      link override pol1_in4_first_tap/sync_delay/Constant3: equ=P=C
  pfb_fir2 : pfb_library/pfb_fir  PFBSize=5  TotalTaps=2  WindowType=hamming  n_inputs=2  MakeBiplex=off  BitWidthIn=8  BitWidthOut=18  CoeffBitWidth=8  CoeffDistMem=off  add_latency=2  mult_latency=3  bram_latency=2  quantization="Round  (unbiased: +/- Inf)"  fwidth=1
      link override pol1_in1_first_tap/sync_delay/Constant: equ=P=C
      link override pol1_in1_first_tap/sync_delay/Constant1: equ=P=C
      link override pol1_in1_first_tap/sync_delay/Constant2: equ=P=C
      link override pol1_in1_first_tap/sync_delay/Constant3: equ=P=C
      link override pol1_in2_first_tap/sync_delay/Constant: equ=P=C
      link override pol1_in2_first_tap/sync_delay/Constant1: equ=P=C
      link override pol1_in2_first_tap/sync_delay/Constant2: equ=P=C
      link override pol1_in2_first_tap/sync_delay/Constant3: equ=P=C
      link override pol1_in3_first_tap/sync_delay/Constant: equ=P=C
      link override pol1_in3_first_tap/sync_delay/Constant1: equ=P=C
      link override pol1_in3_first_tap/sync_delay/Constant2: equ=P=C
      link override pol1_in3_first_tap/sync_delay/Constant3: equ=P=C
      link override pol1_in4_first_tap/sync_delay/Constant: equ=P=C
      link override pol1_in4_first_tap/sync_delay/Constant1: equ=P=C
      link override pol1_in4_first_tap/sync_delay/Constant2: equ=P=C
      link override pol1_in4_first_tap/sync_delay/Constant3: equ=P=C
  pfb_fir3 : pfb_library/pfb_fir  PFBSize=5  TotalTaps=2  WindowType=hamming  n_inputs=2  MakeBiplex=off  BitWidthIn=8  BitWidthOut=18  CoeffBitWidth=8  CoeffDistMem=off  add_latency=2  mult_latency=3  bram_latency=2  quantization="Round  (unbiased: +/- Inf)"  fwidth=1
      link override pol1_in1_first_tap/sync_delay/Constant: equ=P=C
      link override pol1_in1_first_tap/sync_delay/Constant1: equ=P=C
      link override pol1_in1_first_tap/sync_delay/Constant2: equ=P=C
      link override pol1_in1_first_tap/sync_delay/Constant3: equ=P=C
      link override pol1_in2_first_tap/sync_delay/Constant: equ=P=C
      link override pol1_in2_first_tap/sync_delay/Constant1: equ=P=C
      link override pol1_in2_first_tap/sync_delay/Constant2: equ=P=C
      link override pol1_in2_first_tap/sync_delay/Constant3: equ=P=C
      link override pol1_in3_first_tap/sync_delay/Constant: equ=P=C
      link override pol1_in3_first_tap/sync_delay/Constant1: equ=P=C
      link override pol1_in3_first_tap/sync_delay/Constant2: equ=P=C
      link override pol1_in3_first_tap/sync_delay/Constant3: equ=P=C
      link override pol1_in4_first_tap/sync_delay/Constant: equ=P=C
      link override pol1_in4_first_tap/sync_delay/Constant1: equ=P=C
      link override pol1_in4_first_tap/sync_delay/Constant2: equ=P=C
      link override pol1_in4_first_tap/sync_delay/Constant3: equ=P=C
  sync : xbsIndex_r3/Gateway Out  output_type=Double  nbits=8  bin_pt=6  arith_type=Boolean  quantization=Truncate  overflow=Wrap  hdl_port=on  timing_constraint=None  locs_specified=off  LOCs={}  needs_fixed_name=off  show_param=off
      settings: xl_area=[0, 0, 0, 0, 0, 0, 0]
  vacc : correlator_library/vacc  vlen=32/2-6  n_bits=32  bin_pt=0  add_latency=2  arith_type=Unsigned  BitWidthIn=36  BinPtIn=35  streams=6
      link override acc_core/const0: equ=P=C
      link override acc_core/const1: equ=P=C
      link override acc_core/vacc_fifo1/constant: equ=P=C
  wires:
  adc/13 -> pfb_fir/1, pfb_fir2/1
  pfb_fir/1 -> fft/1
  pfb_fir/2 -> fft/3
  pfb_fir/3 -> fft/4
  fft_shift_reg/1 -> fft/2, fft2/2, fft1/2, fft3/2
  Constant/1 -> fft_shift_reg/1
  pfb_fir/4 -> fft/5
  pfb_fir/5 -> fft/6
  adc/1 -> pfb_fir/2
  adc/2 -> pfb_fir/3
  adc/3 -> pfb_fir/4
  adc/4 -> pfb_fir/5
  pfb_fir1/1 -> fft1/1
  pfb_fir1/2 -> fft1/3
  pfb_fir1/3 -> fft1/4
  pfb_fir1/4 -> fft1/5
  pfb_fir1/5 -> fft1/6
  pfb_fir3/1 -> fft3/1
  pfb_fir3/2 -> fft3/3
  pfb_fir3/3 -> fft3/4
  pfb_fir3/4 -> fft3/5
  pfb_fir3/5 -> fft3/6
  adc1/13 -> pfb_fir1/1, pfb_fir3/1
  adc1/1 -> pfb_fir1/2
  adc1/2 -> pfb_fir1/3
  adc1/3 -> pfb_fir1/4
  adc1/4 -> pfb_fir1/5
  adc1/5 -> pfb_fir3/2
  adc1/6 -> pfb_fir3/3
  adc1/7 -> pfb_fir3/4
  adc1/8 -> pfb_fir3/5
  pfb_fir2/1 -> fft2/1
  pfb_fir2/2 -> fft2/3
  pfb_fir2/3 -> fft2/4
  pfb_fir2/4 -> fft2/5
  pfb_fir2/5 -> fft2/6
  adc/5 -> pfb_fir2/2
  adc/6 -> pfb_fir2/3
  adc/7 -> pfb_fir2/4
  adc/8 -> pfb_fir2/5
  Constant1/1 -> adc/4, adc1/4
  fft/2 -> Delay/1
  fft2/2 -> Delay1/1
  fft1/2 -> Delay2/1
  fft3/2 -> Delay12/1
  fft/3 -> Delay3/1
  fft/4 -> Delay4/1
  fft/5 -> Delay5/1
  Mux/1 -> Mult/1, Gateway Out9/1
  Delay/1 -> Mux/2
  Delay3/1 -> Mux/3
  Delay4/1 -> Mux/4
  Delay5/1 -> Mux/5
  mux_sel/1 -> Mux/1, Mux1/1, Mux2/1, Mux3/1, mux select/1
  Delay1/1 -> Mux1/2
  Mux1/1 -> Mult/2, Mult1/1, Mult3/1, Mult4/1, Mult2/1, Gateway Out10/1
  Delay6/1 -> Mux1/3
  Delay7/1 -> Mux1/4
  Delay8/1 -> Mux1/5
  fft2/3 -> Delay6/1
  fft2/4 -> Delay7/1
  fft2/5 -> Delay8/1
  fft3/3 -> Delay13/1
  fft3/4 -> Delay14/1
  fft3/5 -> Delay15/1
  Mux2/1 -> Mult5/1, Mult3/2, Mult1/2, Gateway Out11/1
  Delay12/1 -> Mux3/2
  Delay13/1 -> Mux3/3
  Delay14/1 -> Mux3/4
  Delay15/1 -> Mux3/5
  Mux3/1 -> Mult2/2, Mult4/2, Mult5/2, Gateway Out12/1
  Delay2/1 -> Mux2/2
  Delay9/1 -> Mux2/3
  Delay10/1 -> Mux2/4
  Delay11/1 -> Mux2/5
  fft1/3 -> Delay9/1
  fft1/4 -> Delay10/1
  fft1/5 -> Delay11/1
  Mult/1 -> Concat/1
  Mult1/1 -> Concat/2
  Mult2/1 -> Concat/3
  Mult3/1 -> Concat/4
  Mult4/1 -> Concat/5
  Mult5/1 -> Concat/6
  Delay16/1 -> Counter1/1, Counter2/1
  Convert/1 -> mux_sel/1, Delay16/1
  fft/1 -> Convert/1
  mux select/1 -> Scope1/1
  Gateway Out9/1 -> Scope1/2
  Gateway Out10/1 -> Scope1/3
  Gateway Out11/1 -> Scope1/4
  Gateway Out12/1 -> Scope1/5
  sync/1 -> Scope1/6
  fft3/1 -> sync/1
  Step/1 -> adc/3, adc1/3
  Sine Wave2/1 -> adc1/1
  Sine Wave3/1 -> adc1/2
  Sine Wave/1 -> adc/1
  Sine Wave1/1 -> adc/2
  Counter1/1 -> Relational1/1
  Constant4/1 -> Relational1/2
  Relational1/1 -> vacc/2
  Concat/1 -> vacc/1
  Constant2/1 -> vacc/3
  Relational2/1 -> vacc/4
  Counter2/1 -> Relational2/1
  Constant3/1 -> Relational2/2
